simulink model "TrilaterateBlock"  (R2015a)
settings: Solver=ode45  StartTime=0.0  StopTime=10.0  RelTol=1e-3
InitFcn:
  | Initilization_simulink
values from neighbouring files (symbols this model uses):
  ref = [0 0 0; a0_a1_avg 0 0; xc yc 0]    [set_reference.m]
settings Model: Creator=tzwijger  LastModifiedBy=tzwijger

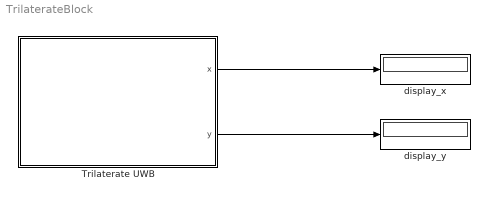
== system TrilaterateBlock ==
  Trilaterate UWB : Subsystem
  display_x : Display
  display_y : Display
  wires:
  Trilaterate UWB/1(x) -> display_x/1
  Trilaterate UWB/2(y) -> display_y/1

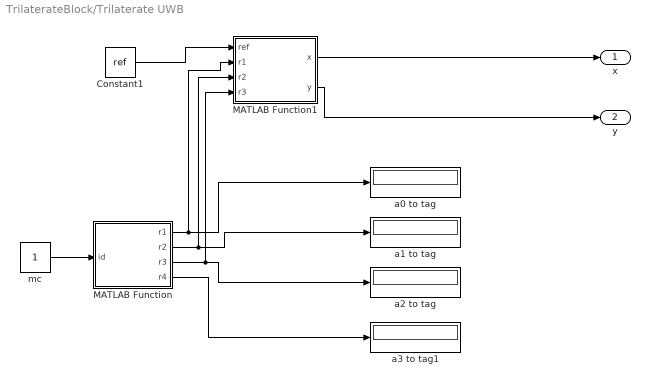
== system TrilaterateBlock/Trilaterate UWB ==
  Constant1 : Constant  Value=ref
  MATLAB Function : MATLAB Function  TreatAsAtomicUnit=on
  MATLAB Function1 : MATLAB Function  TreatAsAtomicUnit=on
  a0 to tag : Display
  a1 to tag : Display
  a2 to tag : Display
  a3 to tag1 : Display
  mc : Constant
  x : Outport
  y : Outport  Port=2
  wires:
  MATLAB Function1/1(x) -> x/1
  MATLAB Function1/2(y) -> y/1
  MATLAB Function/4(r4) -> a3 to tag1/1
  MATLAB Function/1(r1) -> MATLAB Function1/2(r1), a0 to tag/1
  mc/1 -> MATLAB Function/1(id)
  MATLAB Function/2(r2) -> MATLAB Function1/3(r2), a1 to tag/1
  MATLAB Function/3(r3) -> MATLAB Function1/4(r3), a2 to tag/1
  Constant1/1 -> MATLAB Function1/1(ref)

== matlab function TrilaterateBlock/Trilaterate UWB/MATLAB Function1 ==
  data: x output; ref input; y output; r1 input; r2 input; r3 input
function [x,y] = trilateration(ref,r1,r2,r3)
persistent plots k fign field2im_params nrplots
if isempty(plots)
    plots = [];
    k = 1;
    load('PlotVars.mat')
end

P = Trilateration(ref',[r1 r2 r3],eye(3));

% Plot and print results
[plots, k] = update_plot_trilat(plots, k, fign, P(2:3), field2im_params, nrplots);

x = P(2);
y = P(3);

== matlab function TrilaterateBlock/Trilaterate UWB/MATLAB Function ==
  data: id input; r1 output; r2 output; r3 output; r4 output
function [r1,r2,r3,r4] = GetMC_sm(id) 
    % Input: Serial Port to A0
    %        
    % Output: Raw data for triangulation
    %
    % Message syntax is explained in the Decawave documentation
    % DecaRangeRTLS_PC_Source_Code_Guide.pdf  - Section 2.3.2
    % DecaRangeRTLS_ARM_Source_Code_Guide.pdf - Section 2.6

    % Make sure to get a measurement with the correct identifier
    persistent s;
    %coder.extrinsic('instrfind','delete','serial','fscanf','strsplit')
    coder.extrinsic('instrfind','delete','serial','fscanf','GetMC')
    
    r1 = 0; r2 = 0; r3 = 0; r4 = 0;
    
    if isempty(s)
        ports = instrfind;
        if ~isempty(ports)
            fclose(ports);
            delete(ports);
        end
        % Establish new connection
        s = serial('COM33','BaudRate',9600,'Parity','None');

        % Open connection
        fopen(s);
        fscanf(s); % Get init mc out of the way and test connection
    end
    
    ids = ['mc';'mr';'ma'];
    id = ids(id,:);
    
    dist = zeros(1,4);
    dist = GetMC(s,id);
    r1 = dist(1);
    r2 = dist(2);
    r3 = dist(3);
    r4 = dist(4); 
end
